simulink model "Q6aug"  (R2018a)
settings: Solver=VariableStepAuto  StartTime=0.0  StopTime=2  RelTol=1e-3
values from neighbouring files (symbols this model uses):
  A = [0.110571547291 0.471247754055 0.0249955131485 2.58943408161e-06 -0.326108592505 0.861622655316 0.0987425683373 1.02293307698e-05 -0.0747829687831 -0.0317325850518 0.998316867847 0.000207017546418 ... (16 elements, 4x4)]    [Q6.mat]    (also in SteelMillControl10.m = DiscPlant.A; SteelMillControl11.m = DiscPlant.A; SteelMillControl12.m = DiscPlant.A; SteelMillControl12lqr.m = DiscPlant.A)
  B = [0.00184081153928 0.000781109785891 4.14309453057e-05 4.29207838905e-09]    [Q6.mat]    (also in SteelMillControl10.m = DiscPlant.B; SteelMillControl11.m = DiscPlant.B; SteelMillControl12.m = DiscPlant.B; SteelMillControl12lqr.m = DiscPlant.B)
  C = [6.47358520402e-07 2.55733269246e-06 5.17543866044e-05 0.5]    [Q6.mat]    (also in SteelMillControl10.m = DiscPlant.C; SteelMillControl11.m = DiscPlant.C; SteelMillControl12.m = DiscPlant.C; SteelMillControl12lqr.m = DiscPlant.C)
  h = 9    [OlaSoup.m]    (also in Q3.mat = 0.0153022172533; Q6.mat = 0.03257469729; Q9disc.mat = 0.532796640949; SteelMillControl11.m = stepRes.RiseTime/11)
  K = [378.478532375 741.649236937 3450.29104505 3374760.11938]    [Q6.mat]    (also in SteelMillControl10.m = place(A,B,dp); SteelMillControl12.m = place(A,B,dp); SteelMillControl5.m = place(A,B,dp); SteelMillControl6.m = place(A,B,dp))
  L = (place(A',C',dp/1.5))'    [SteelMillControl6.m]    (also in SteelMillControl6aug.m)
  Lcorr = inv(dcgain(ss(A-B*K,B,C,D,h)))    [SteelMillControl10.m]    (also in SteelMillControl11.m; SteelMillControl12.m; SteelMillControl12lqr.m; SteelMillControl5.m)
  xinit = [-17 5 -8 0.5]    [Q6.mat]    (also in SteelMillControl10.m = [0 0 0 0]; SteelMillControl11.m = [0 0 0 0]; SteelMillControl12.m = [0 0 0 0]; SteelMillControl12lqr.m = [0 0 0 0])
  xinitObs = [0 0 0 0]    [Q6.mat]    (also in SteelMillControl6.m; SteelMillControl6aug.m = [xinitObs 0])
settings Model: Creator=bakos  LastModifiedBy=bakos
settings SolverCC: DecoupledContinuousIntegration=on  MinimalZcImpactIntegration=on

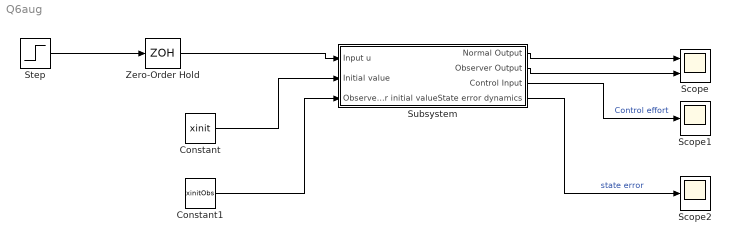
== system Q6aug ==
  Constant : Constant  Value=xinit
  Constant1 : Constant  Value=xinitObs
  Scope : Scope  NumInputPorts=2
  Scope1 : Scope
  Scope2 : Scope
  Step : Step  Time=0  SampleTime=0
  Subsystem : Subsystem
  Zero-Order Hold : ZeroOrderHold  SampleTime=h
  wires:
  Subsystem/3(Control Input) -> Scope1/1  "Control effort"
  Subsystem/1(Normal Output) -> Scope/1
  Subsystem/2(Observer Output) -> Scope/2
  Step/1 -> Zero-Order Hold/1
  Constant1/1 -> Subsystem/3(Observer initial value)
  Subsystem/4(State error dynamics) -> Scope2/1  "state error"
  Constant/1 -> Subsystem/2(Initial value)
  Zero-Order Hold/1 -> Subsystem/1(Input u)

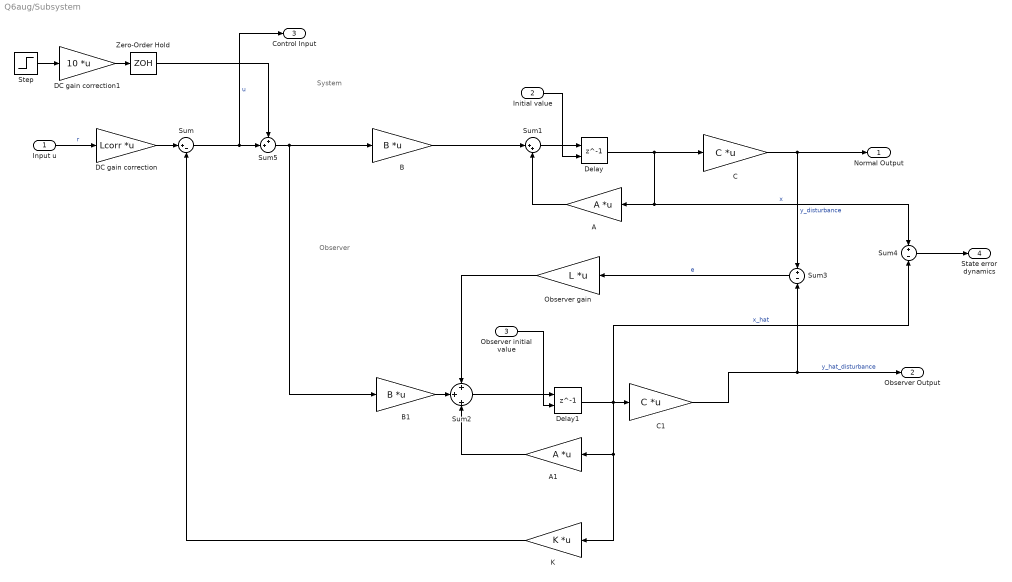
== system Q6aug/Subsystem ==
  note: System
  note: Observer
  Input u : Inport
  Initial value : Inport  Port=2
  Observer initial value : Inport  Port=3
  A : Gain  Gain=A  Multiplication=Matrix(K*u)
  A1 : Gain  Gain=A  Multiplication=Matrix(K*u)
  B : Gain  Gain=B  Multiplication=Matrix(K*u)
  B1 : Gain  Gain=B  Multiplication=Matrix(K*u)
  C : Gain  Gain=C  Multiplication=Matrix(K*u)
  C1 : Gain  Gain=C  Multiplication=Matrix(K*u)
  DC gain correction : Gain  Gain=Lcorr  Multiplication=Matrix(K*u)
  DC gain correction1 : Gain  Gain=10  Multiplication=Matrix(K*u)
  Delay : Delay  DelayLength=1  InitialConditionSource=Input port  InitialCondition=0  SampleTime=h
      settings: InputPortMap=u0,p4
  Delay1 : Delay  DelayLength=1  InitialConditionSource=Input port  SampleTime=h
      settings: InputPortMap=u0,p4
  K : Gain  Gain=K  Multiplication=Matrix(K*u)
  Observer gain : Gain  Gain=L  Multiplication=Matrix(K*u)
  Step : Step  SampleTime=0
  Sum : Sum  Inputs=|+-
  Sum1 : Sum  Inputs=|++
  Sum2 : Sum  Inputs=+|+|+
  Sum3 : Sum  Inputs=+|-
  Sum4 : Sum  Inputs=+|-
  Sum5 : Sum  Inputs=++|
  Zero-Order Hold : ZeroOrderHold  SampleTime=h
  Normal Output : Outport
  Observer Output : Outport  Port=2
  Control Input : Outport  Port=3
  State error dynamics : Outport  Port=4
  wires:
  Sum/1 -> Sum5/2, Control Input/1  "u"
  B/1 -> Sum1/1
  Sum1/1 -> Delay/1
  Delay/1 -> Sum4/1, A/1, C/1  "x"
  C/1 -> Sum3/1, Normal Output/1  "y_disturbance"
  A/1 -> Sum1/2
  C1/1 -> Observer Output/1, Sum3/2  "y_hat_disturbance"
  Delay1/1 -> Sum4/2, C1/1, K/1, A1/1  "x_hat"
  Input u/1 -> DC gain correction/1  "r"
  Sum2/1 -> Delay1/1
  Initial value/1 -> Delay/2
  Observer initial value/1 -> Delay1/2
  A1/1 -> Sum2/3
  B1/1 -> Sum2/2
  Observer gain/1 -> Sum2/1
  Sum3/1 -> Observer gain/1  "e"
  Step/1 -> DC gain correction1/1
  DC gain correction1/1 -> Zero-Order Hold/1
  Sum4/1 -> State error dynamics/1
  Zero-Order Hold/1 -> Sum5/1
  Sum5/1 -> B1/1, B/1
  DC gain correction/1 -> Sum/1
  K/1 -> Sum/2
